simulink model "secorderpid2nd_2016"  (R2016b)
settings: Solver=ode23  StartTime=0.0  StopTime=30  FixedStep=1e-3  MaxStep=5e-4  RelTol=5e-4
values from neighbouring files (symbols this model uses):
  b = [1 0]    [Exemple_2_disertacao.mat]    (also in Lpid.m = j*w(a); example_result_gasearch_nelson_com_PID.mat = [0 0 1 1])
  C = [1  -0.9999; -0.9999  1]    [Exemple_2_disertacao.mat]    (also in example2MG.mat = [0.5 0 0 0 0 0 0 0 0 0 0 0 ... (16 elements, 4x4)]; example_result_gasearch_nelson_com_PID.mat = [0.5 0 -0.5 0 0 0 0 0 -0.5 0 0.5 0 ... (16 elements, 4x4)]; wingcons.mat = [7.66  2.45  2.1; 0.23  1.04  0.223; 0.6  0.756  0.658])
  d = [1 0]    [Exemple_2_disertacao.mat]    (also in Exemple_6_disertacao.mat; example2MG.mat = [1 6 15 18 10]; example_result_gasearch_nelson_com_PID.mat = [0 0 1 1])
  dx0 = [0 0]    [Exemple_2_disertacao.mat]    (also in Exemple_6_disertacao.mat; example2MG.mat = [0 0 0 0])
  K = [2.5 -1 0 0 0 0 0 0 0 0 0 0 ... (2500 elements, 50x50)]    [Belloti_N50.mat]    (also in Exemple_2_disertacao.mat = [3  -2; -2  3]; Exemple_6_disertacao.mat = [3  -2; -2  3]; example2MG.mat = [5 -5 0 0 -5 10 -5 0 0 -5 10 -5 ... (16 elements, 4x4)]; example_result_gasearch_nelson_com_PID.mat = [200 0 -100 0 0 200 0 -100 -100 0 150 -50 ... (16 elements, )
  M = [4 0 0 0 0 0 0 0 0 0 0 0 ... (2500 elements, 50x50)]    [Belloti_N50.mat]    (also in Exemple_2_disertacao.mat = [1  0; 0  1]; Exemple_6_disertacao.mat = [1  0; 0  1]; example2MG.mat = [1 0 0 0 0 1 0 0 0 0 1 0 ... (16 elements, 4x4)]; example_result_gasearch_nelson_com_PID.mat = [1 0 0 0 0 1 0 0 0 0 1 0 ... (16 elements, 4x4)])
  tau = 0.1    [Belloti_N50.mat]    (also in Exemple_2_disertacao.mat = 0.5; Exemple_6_disertacao.mat = 0.5; example_result_gasearch_nelson_com_PID.mat = 0.05)
  x0 = [1 0 0 0 0 0 0 0 0 0 0 0 ... (50 elements, 1x50)]    [Belloti_N50.mat]    (also in Exemple_2_disertacao.mat = [0 0]; Exemple_6_disertacao.mat = [0 0]; example2MG.mat = [0 0 0 0]; example_result_gasearch_nelson_com_PID.mat = [1 0 0 0])
settings Model: Creator=Jose  LastModifiedBy=jhona
settings DataIOCC: LimitDataPoints=on  SaveFormat=Array  SignalLoggingSaveFormat=ModelDataLogs
settings OptimizationCC: BlockReduction=off  BooleanDataType=off  ExpressionDepthLimit=2147483647  EfficientMapNaN2IntZero=off  LifeSpan=inf
settings DebuggingCC: SaveWithParameterizedLinksMsg=none  UnderspecifiedInitializationDetection=Classic  MergeDetectMultiDrivingBlocksExec=none  SignalResolutionControl=TryResolveAllWithWarning  MultiTaskDSMMsg=warning  MultiTaskCondExecSysMsg=none  StateNameClashWarn=warning  SFUnexpectedBacktrackingDiag=warning  SFNoUnconditionalDefaultTransitionDiag=warning  SFExecutionAtInitializationDiag=none
settings HardwareCC: ProdBitPerPointer=32  ProdBitPerSizeT=32  ProdBitPerPtrDiffT=32  ProdLargestAtomicFloat=None  ProdIntDivRoundTo=Undefined  ProdEndianess=Unspecified  ProdWordSize=32  ProdHWDeviceType=32-bit Generic  TargetBitPerPointer=64  TargetBitPerSizeT=64  TargetBitPerPtrDiffT=64  TargetLongLongMode=on  TargetIntDivRoundTo=Zero  TargetEndianess=LittleEndian  TargetWordSize=64  TargetHWDeviceType=MATLAB Host  ProdEqTarget=off
settings ModelReferenceCC: PropagateSignalLabelsOutOfModel=off
settings CodeAppCC: MaxIdLength=128
settings GRTTargetCC: TargetLangStandard=C89/C90 (ANSI)  CombineOutputUpdateFcns=off  GRTInterface=on
settings ConfigComp: CovMetricSettings=dw  CovHtmlReporting=on  CovSaveCumulativeToWorkspaceVar=on  CovSaveSingleToWorkspaceVar=on  CovExternalEMLEnable=off

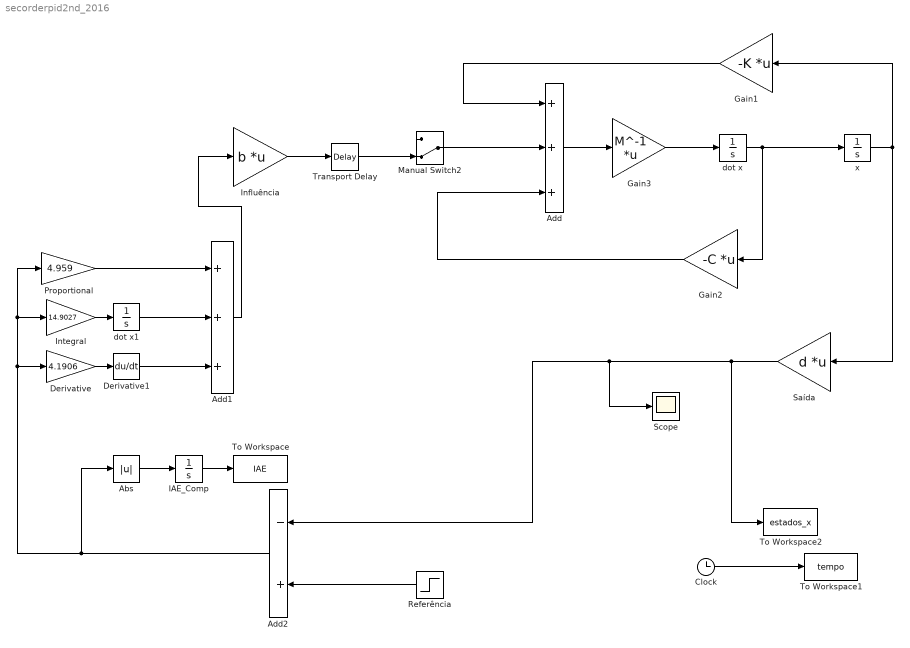
== system secorderpid2nd_2016 ==
  Abs : Abs
  Add : Sum  Inputs=+++
  Add1 : Sum  Inputs=+++
  Add2 : Sum  Inputs=-+
  Clock : Clock
  Derivative : Gain  Gain=4.1906
  Derivative1 : Derivative  CoefficientInTFapproximation=100
  Gain1 : Gain  Gain=-K  Multiplication=Matrix(K*u)
  Gain2 : Gain  Gain=-C  Multiplication=Matrix(K*u)
  Gain3 : Gain  Gain=M^-1  Multiplication=Matrix(K*u)
  IAE_Comp : Integrator
  Influência : Gain  Gain=b  Multiplication=Matrix(K*u)
  Integral : Gain  Gain=14.9027
  Manual Switch2 : ManualSwitch  CurrentSetting=0
  Proportional : Gain  Gain=4.959
  Referência : Step  Time=0  SampleTime=0
  Saída : Gain  Gain=d  Multiplication=Matrix(K*u)
  Scope : Scope
  To Workspace : ToWorkspace  VariableName=IAE  SampleTime=-1
  To Workspace1 : ToWorkspace  VariableName=tempo  SampleTime=-1
  To Workspace2 : ToWorkspace  VariableName=estados_x  SampleTime=-1
  Transport Delay : TransportDelay  DelayTime=tau  BufferSize=2048
  dot x : Integrator  InitialCondition=dx0
  dot x1 : Integrator
  x : Integrator  InitialCondition=x0
  wires:
  Gain1/1 -> Add/1
  Add/1 -> Gain3/1
  Gain3/1 -> dot x/1
  dot x/1 -> Gain2/1, x/1
  Gain2/1 -> Add/3
  Influência/1 -> Transport Delay/1
  Manual Switch2/1 -> Add/2
  Transport Delay/1 -> Manual Switch2/2
  Proportional/1 -> Add1/1
  Integral/1 -> dot x1/1
  dot x1/1 -> Add1/2
  Derivative1/1 -> Add1/3
  Derivative/1 -> Derivative1/1
  Referência/1 -> Add2/2
  Add1/1 -> Influência/1
  Add2/1 -> Abs/1, Proportional/1, Integral/1, Derivative/1
  Abs/1 -> IAE_Comp/1
  IAE_Comp/1 -> To Workspace/1
  Clock/1 -> To Workspace1/1
  x/1 -> Saída/1, Gain1/1
  Saída/1 -> To Workspace2/1, Scope/1, Add2/1
